simulink model "gm_uz_pmsm_model_9ph_21b_all_double_vnl"  (R2021b)
settings: Solver=FixedStepDiscrete  StartTime=0.0  StopTime=0.8  RelTol=1e-3
PreLoadFcn:
  | uz_pmsm_model_9ph_init_parameter
undefined symbols (not defined in the file or in its folder): a, b, c, friction_coefficient, inertia, k_i_d, k_i_q, k_p_d, k_p_q, Kpd, L_d, L_o1, L_o2, L_q, L_x1, L_x2, L_y1, L_y2, L_zero, polepair, psi_pm, R_1, static_friction_torque, Tnd, ts
libraries: hdlmdlgenlib x139, hdlsllib x90, dspsigops x21, simulink x17, slpidlib x2, spsAlphaBetaZerotodq0Lib x1, pid_lib x1, spsdq0toAlphaBetaZeroLib x1
(part 4 of 5)

== system gm_uz_pmsm_model_9ph_21b_all_double_vnl/uz_pmsm_model_9ph/Line-Line to Phase voltage/abc   to   alpha_beta_0 ==
  "a, b, c" : Inport  OutDataTypeStr=fixdt(1, 25, 12)  PortDimensions=[3]  SampleTime=1e-08
  Gain2 : Product  Inputs=**  OutDataTypeStr=fixdt(1, 43, 28)  SampleTime=1e-08
  Gain2_const : Constant  Value=0.6666717529296875  OutDataTypeStr=fixdt(1, 18, 16)  SampleTime=1e-08
  Gain2_out_dtc : DataTypeConversion  OutDataTypeStr=fixdt(1, 25, 12)  SampleTime=1e-08  SaturateOnIntegerOverflow=on
  Gain4_const : Constant  Value=[1;0;0.5;-0.5;0.86602783203125;0.5;-0.5;-0.86602783203125;0.5]  OutDataTypeStr=fixdt(1, 18, 16)  SampleTime=1e-08
  HwModeRegister{,1..3} (4 alike) : Delay  DelayLength=double(1)  InitialCondition=0  SampleTime=1e-08
  MMul_add_01 : Sum  OutDataTypeStr=fixdt(1, 25, 12)  SaturateOnIntegerOverflow=on  SampleTime=1e-08
  MMul_add_12 : Sum  OutDataTypeStr=fixdt(1, 25, 12)  SaturateOnIntegerOverflow=on  SampleTime=1e-08
  MMul_dot_product : Product  Inputs=**  OutDataTypeStr=fixdt(1, 43, 28)  SampleTime=1e-08
  MMul_dot_product_out_dtc : DataTypeConversion  OutDataTypeStr=fixdt(1, 25, 12)  SampleTime=1e-08  SaturateOnIntegerOverflow=on
  PipelineRegister : Delay  DelayLength=double(1)  InitialCondition=0  SampleTime=1e-08
  PipelineRegister1 : Delay  DelayLength=double(1)  InitialCondition=0  SampleTime=1e-08
  Reshape : Reshape  OutputDimensionality=Column vector (2-D)
  Row2Col_in0 : Reshape  OutputDimensionality=Column vector (2-D)
  Row2Col_in1 : Reshape  OutputDimensionality=Column vector (2-D)
  reshape_dotProduct : Reshape  OutputDimensionality=Customize  OutputDimensions=[3,3]
  reshape_mmulResult : Reshape  OutputDimensionality=Customize  OutputDimensions=[3,1]
  select_0 : Selector  NumberOfDimensions=2  SampleTime=1e-08  IndexOptions=Index vector (dialog),Select all  Indices=double(1),[]  OutputSizes=1
  select_1 : Selector  NumberOfDimensions=2  SampleTime=1e-08  IndexOptions=Index vector (dialog),Select all  Indices=double(2),[]  OutputSizes=1
  select_2 : Selector  NumberOfDimensions=2  SampleTime=1e-08  IndexOptions=Index vector (dialog),Select all  Indices=double(3),[]  OutputSizes=1
  select_indices0 : Selector  SampleTime=1e-08  IndexOptions=Index vector (dialog)  Indices=double([1 4 7 2 5 8 3 6 9])  OutputSizes=1
  select_indices1 : Selector  SampleTime=1e-08  IndexOptions=Index vector (dialog)  Indices=double([1 2 3 1 2 3 1 2 3])  OutputSizes=1
  t : Reshape  OutputDimensionality=Customize  OutputDimensions=[3,3]
  vectorized_in0 : Reshape  OutputDimensionality=Row vector (2-D)
  "alpha, beta, 0 " : Outport  SampleTime=1e-08
  wires:
  HwModeRegister3/1 -> Gain2/2
  HwModeRegister2/1 -> Gain2/1
  Gain2/1 -> PipelineRegister1/1
  HwModeRegister1/1 -> MMul_dot_product/2
  HwModeRegister/1 -> MMul_dot_product/1
  MMul_dot_product/1 -> PipelineRegister/1
  "a, b, c"/1 -> Reshape/1
  PipelineRegister1/1 -> Gain2_out_dtc/1
  PipelineRegister/1 -> MMul_dot_product_out_dtc/1
  Gain2_const/1 -> HwModeRegister3/1
  Gain4_const/1 -> t/1
  MMul_add_12/1 -> reshape_mmulResult/1
  select_2/1 -> MMul_add_12/2
  MMul_add_01/1 -> MMul_add_12/1
  select_1/1 -> MMul_add_01/2
  select_0/1 -> MMul_add_01/1
  reshape_dotProduct/1 -> select_0/1, select_1/1, select_2/1
  MMul_dot_product_out_dtc/1 -> reshape_dotProduct/1
  Row2Col_in1/1 -> HwModeRegister1/1
  Row2Col_in0/1 -> HwModeRegister/1
  select_indices1/1 -> Row2Col_in1/1
  select_indices0/1 -> Row2Col_in0/1
  vectorized_in0/1 -> select_indices0/1
  t/1 -> vectorized_in0/1
  Reshape/1 -> select_indices1/1
  reshape_mmulResult/1 -> HwModeRegister2/1
  Gain2_out_dtc/1 -> "alpha, beta, 0 "/1

== system gm_uz_pmsm_model_9ph_21b_all_double_vnl/uz_pmsm_model_9ph/Line-Line to Phase voltage/alpha_beta_0   to   abc ==
  "alpha, beta, 0  " : Inport  OutDataTypeStr=fixdt(1, 25, 12)  PortDimensions=[3]  SampleTime=1e-08
  Gain4_const : Constant  Value=[1;-0.5;-0.5;0;0.86602783203125;-0.86602783203125;1;1;1]  OutDataTypeStr=fixdt(1, 18, 16)  SampleTime=1e-08
  HwModeRegister : Delay  DelayLength=double(1)  InitialCondition=0  SampleTime=1e-08
  HwModeRegister1 : Delay  DelayLength=double(1)  InitialCondition=0  SampleTime=1e-08
  MMul_add_01 : Sum  OutDataTypeStr=fixdt(1, 25, 12)  SaturateOnIntegerOverflow=on  SampleTime=1e-08
  MMul_add_12 : Sum  OutDataTypeStr=fixdt(1, 25, 12)  SaturateOnIntegerOverflow=on  SampleTime=1e-08
  MMul_dot_product : Product  Inputs=**  OutDataTypeStr=fixdt(1, 43, 28)  SampleTime=1e-08
  MMul_dot_product_out_dtc : DataTypeConversion  OutDataTypeStr=fixdt(1, 25, 12)  SampleTime=1e-08  SaturateOnIntegerOverflow=on
  PipelineRegister : Delay  DelayLength=double(1)  InitialCondition=0  SampleTime=1e-08
  Reshape : Reshape  OutputDimensionality=Column vector (2-D)
  Row2Col_in0 : Reshape  OutputDimensionality=Column vector (2-D)
  Row2Col_in1 : Reshape  OutputDimensionality=Column vector (2-D)
  reshape_dotProduct : Reshape  OutputDimensionality=Customize  OutputDimensions=[3,3]
  reshape_mmulResult : Reshape  OutputDimensionality=Customize  OutputDimensions=[3,1]
  select_0 : Selector  NumberOfDimensions=2  SampleTime=1e-08  IndexOptions=Index vector (dialog),Select all  Indices=double(1),[]  OutputSizes=1
  select_1 : Selector  NumberOfDimensions=2  SampleTime=1e-08  IndexOptions=Index vector (dialog),Select all  Indices=double(2),[]  OutputSizes=1
  select_2 : Selector  NumberOfDimensions=2  SampleTime=1e-08  IndexOptions=Index vector (dialog),Select all  Indices=double(3),[]  OutputSizes=1
  select_indices0 : Selector  SampleTime=1e-08  IndexOptions=Index vector (dialog)  Indices=double([1 4 7 2 5 8 3 6 9])  OutputSizes=1
  select_indices1 : Selector  SampleTime=1e-08  IndexOptions=Index vector (dialog)  Indices=double([1 2 3 1 2 3 1 2 3])  OutputSizes=1
  t : Reshape  OutputDimensionality=Customize  OutputDimensions=[3,3]
  vectorized_in0 : Reshape  OutputDimensionality=Row vector (2-D)
  "a, b, c" : Outport  SampleTime=1e-08
  wires:
  HwModeRegister1/1 -> MMul_dot_product/2
  HwModeRegister/1 -> MMul_dot_product/1
  MMul_dot_product/1 -> PipelineRegister/1
  "alpha, beta, 0  "/1 -> Reshape/1
  PipelineRegister/1 -> MMul_dot_product_out_dtc/1
  Gain4_const/1 -> t/1
  MMul_add_12/1 -> reshape_mmulResult/1
  select_2/1 -> MMul_add_12/2
  MMul_add_01/1 -> MMul_add_12/1
  select_1/1 -> MMul_add_01/2
  select_0/1 -> MMul_add_01/1
  reshape_dotProduct/1 -> select_0/1, select_1/1, select_2/1
  MMul_dot_product_out_dtc/1 -> reshape_dotProduct/1
  Row2Col_in1/1 -> HwModeRegister1/1
  Row2Col_in0/1 -> HwModeRegister/1
  select_indices1/1 -> Row2Col_in1/1
  select_indices0/1 -> Row2Col_in0/1
  vectorized_in0/1 -> select_indices0/1
  t/1 -> vectorized_in0/1
  Reshape/1 -> select_indices1/1
  reshape_mmulResult/1 -> "a, b, c"/1

== system gm_uz_pmsm_model_9ph_21b_all_double_vnl/uz_pmsm_model_9ph/Line-Line to Phase voltage1/abc   to   alpha_beta_0 ==
  "a, b, c" : Inport  OutDataTypeStr=fixdt(1, 25, 12)  PortDimensions=[3]  SampleTime=1e-08
  Gain2 : Product  Inputs=**  OutDataTypeStr=fixdt(1, 43, 28)  SampleTime=1e-08
  Gain2_const : Constant  Value=0.6666717529296875  OutDataTypeStr=fixdt(1, 18, 16)  SampleTime=1e-08
  Gain2_out_dtc : DataTypeConversion  OutDataTypeStr=fixdt(1, 25, 12)  SampleTime=1e-08  SaturateOnIntegerOverflow=on
  Gain4_const : Constant  Value=[1;0;0.5;-0.5;0.86602783203125;0.5;-0.5;-0.86602783203125;0.5]  OutDataTypeStr=fixdt(1, 18, 16)  SampleTime=1e-08
  HwModeRegister{,1..3} (4 alike) : Delay  DelayLength=double(1)  InitialCondition=0  SampleTime=1e-08
  MMul_add_01 : Sum  OutDataTypeStr=fixdt(1, 25, 12)  SaturateOnIntegerOverflow=on  SampleTime=1e-08
  MMul_add_12 : Sum  OutDataTypeStr=fixdt(1, 25, 12)  SaturateOnIntegerOverflow=on  SampleTime=1e-08
  MMul_dot_product : Product  Inputs=**  OutDataTypeStr=fixdt(1, 43, 28)  SampleTime=1e-08
  MMul_dot_product_out_dtc : DataTypeConversion  OutDataTypeStr=fixdt(1, 25, 12)  SampleTime=1e-08  SaturateOnIntegerOverflow=on
  PipelineRegister : Delay  DelayLength=double(1)  InitialCondition=0  SampleTime=1e-08
  PipelineRegister1 : Delay  DelayLength=double(1)  InitialCondition=0  SampleTime=1e-08
  Reshape : Reshape  OutputDimensionality=Column vector (2-D)
  Row2Col_in0 : Reshape  OutputDimensionality=Column vector (2-D)
  Row2Col_in1 : Reshape  OutputDimensionality=Column vector (2-D)
  reshape_dotProduct : Reshape  OutputDimensionality=Customize  OutputDimensions=[3,3]
  reshape_mmulResult : Reshape  OutputDimensionality=Customize  OutputDimensions=[3,1]
  select_0 : Selector  NumberOfDimensions=2  SampleTime=1e-08  IndexOptions=Index vector (dialog),Select all  Indices=double(1),[]  OutputSizes=1
  select_1 : Selector  NumberOfDimensions=2  SampleTime=1e-08  IndexOptions=Index vector (dialog),Select all  Indices=double(2),[]  OutputSizes=1
  select_2 : Selector  NumberOfDimensions=2  SampleTime=1e-08  IndexOptions=Index vector (dialog),Select all  Indices=double(3),[]  OutputSizes=1
  select_indices0 : Selector  SampleTime=1e-08  IndexOptions=Index vector (dialog)  Indices=double([1 4 7 2 5 8 3 6 9])  OutputSizes=1
  select_indices1 : Selector  SampleTime=1e-08  IndexOptions=Index vector (dialog)  Indices=double([1 2 3 1 2 3 1 2 3])  OutputSizes=1
  t : Reshape  OutputDimensionality=Customize  OutputDimensions=[3,3]
  vectorized_in0 : Reshape  OutputDimensionality=Row vector (2-D)
  "alpha, beta, 0 " : Outport  SampleTime=1e-08
  wires:
  HwModeRegister3/1 -> Gain2/2
  HwModeRegister2/1 -> Gain2/1
  Gain2/1 -> PipelineRegister1/1
  HwModeRegister1/1 -> MMul_dot_product/2
  HwModeRegister/1 -> MMul_dot_product/1
  MMul_dot_product/1 -> PipelineRegister/1
  "a, b, c"/1 -> Reshape/1
  PipelineRegister1/1 -> Gain2_out_dtc/1
  PipelineRegister/1 -> MMul_dot_product_out_dtc/1
  Gain2_const/1 -> HwModeRegister3/1
  Gain4_const/1 -> t/1
  MMul_add_12/1 -> reshape_mmulResult/1
  select_2/1 -> MMul_add_12/2
  MMul_add_01/1 -> MMul_add_12/1
  select_1/1 -> MMul_add_01/2
  select_0/1 -> MMul_add_01/1
  reshape_dotProduct/1 -> select_0/1, select_1/1, select_2/1
  MMul_dot_product_out_dtc/1 -> reshape_dotProduct/1
  Row2Col_in1/1 -> HwModeRegister1/1
  Row2Col_in0/1 -> HwModeRegister/1
  select_indices1/1 -> Row2Col_in1/1
  select_indices0/1 -> Row2Col_in0/1
  vectorized_in0/1 -> select_indices0/1
  t/1 -> vectorized_in0/1
  Reshape/1 -> select_indices1/1
  reshape_mmulResult/1 -> HwModeRegister2/1
  Gain2_out_dtc/1 -> "alpha, beta, 0 "/1

== system gm_uz_pmsm_model_9ph_21b_all_double_vnl/uz_pmsm_model_9ph/Line-Line to Phase voltage1/alpha_beta_0   to   abc ==
  "alpha, beta, 0  " : Inport  OutDataTypeStr=fixdt(1, 25, 12)  PortDimensions=[3]  SampleTime=1e-08
  Gain4_const : Constant  Value=[1;-0.5;-0.5;0;0.86602783203125;-0.86602783203125;1;1;1]  OutDataTypeStr=fixdt(1, 18, 16)  SampleTime=1e-08
  HwModeRegister : Delay  DelayLength=double(1)  InitialCondition=0  SampleTime=1e-08
  HwModeRegister1 : Delay  DelayLength=double(1)  InitialCondition=0  SampleTime=1e-08
  MMul_add_01 : Sum  OutDataTypeStr=fixdt(1, 25, 12)  SaturateOnIntegerOverflow=on  SampleTime=1e-08
  MMul_add_12 : Sum  OutDataTypeStr=fixdt(1, 25, 12)  SaturateOnIntegerOverflow=on  SampleTime=1e-08
  MMul_dot_product : Product  Inputs=**  OutDataTypeStr=fixdt(1, 43, 28)  SampleTime=1e-08
  MMul_dot_product_out_dtc : DataTypeConversion  OutDataTypeStr=fixdt(1, 25, 12)  SampleTime=1e-08  SaturateOnIntegerOverflow=on
  PipelineRegister : Delay  DelayLength=double(1)  InitialCondition=0  SampleTime=1e-08
  Reshape : Reshape  OutputDimensionality=Column vector (2-D)
  Row2Col_in0 : Reshape  OutputDimensionality=Column vector (2-D)
  Row2Col_in1 : Reshape  OutputDimensionality=Column vector (2-D)
  reshape_dotProduct : Reshape  OutputDimensionality=Customize  OutputDimensions=[3,3]
  reshape_mmulResult : Reshape  OutputDimensionality=Customize  OutputDimensions=[3,1]
  select_0 : Selector  NumberOfDimensions=2  SampleTime=1e-08  IndexOptions=Index vector (dialog),Select all  Indices=double(1),[]  OutputSizes=1
  select_1 : Selector  NumberOfDimensions=2  SampleTime=1e-08  IndexOptions=Index vector (dialog),Select all  Indices=double(2),[]  OutputSizes=1
  select_2 : Selector  NumberOfDimensions=2  SampleTime=1e-08  IndexOptions=Index vector (dialog),Select all  Indices=double(3),[]  OutputSizes=1
  select_indices0 : Selector  SampleTime=1e-08  IndexOptions=Index vector (dialog)  Indices=double([1 4 7 2 5 8 3 6 9])  OutputSizes=1
  select_indices1 : Selector  SampleTime=1e-08  IndexOptions=Index vector (dialog)  Indices=double([1 2 3 1 2 3 1 2 3])  OutputSizes=1
  t : Reshape  OutputDimensionality=Customize  OutputDimensions=[3,3]
  vectorized_in0 : Reshape  OutputDimensionality=Row vector (2-D)
  "a, b, c" : Outport  SampleTime=1e-08
  wires:
  HwModeRegister1/1 -> MMul_dot_product/2
  HwModeRegister/1 -> MMul_dot_product/1
  MMul_dot_product/1 -> PipelineRegister/1
  "alpha, beta, 0  "/1 -> Reshape/1
  PipelineRegister/1 -> MMul_dot_product_out_dtc/1
  Gain4_const/1 -> t/1
  MMul_add_12/1 -> reshape_mmulResult/1
  select_2/1 -> MMul_add_12/2
  MMul_add_01/1 -> MMul_add_12/1
  select_1/1 -> MMul_add_01/2
  select_0/1 -> MMul_add_01/1
  reshape_dotProduct/1 -> select_0/1, select_1/1, select_2/1
  MMul_dot_product_out_dtc/1 -> reshape_dotProduct/1
  Row2Col_in1/1 -> HwModeRegister1/1
  Row2Col_in0/1 -> HwModeRegister/1
  select_indices1/1 -> Row2Col_in1/1
  select_indices0/1 -> Row2Col_in0/1
  vectorized_in0/1 -> select_indices0/1
  t/1 -> vectorized_in0/1
  Reshape/1 -> select_indices1/1
  reshape_mmulResult/1 -> "a, b, c"/1

== system gm_uz_pmsm_model_9ph_21b_all_double_vnl/uz_pmsm_model_9ph/Line-Line to Phase voltage2/abc   to   alpha_beta_0 ==
  "a, b, c" : Inport  OutDataTypeStr=fixdt(1, 25, 12)  PortDimensions=[3]  SampleTime=1e-08
  Gain2 : Product  Inputs=**  OutDataTypeStr=fixdt(1, 43, 28)  SampleTime=1e-08
  Gain2_const : Constant  Value=0.6666717529296875  OutDataTypeStr=fixdt(1, 18, 16)  SampleTime=1e-08
  Gain2_out_dtc : DataTypeConversion  OutDataTypeStr=fixdt(1, 25, 12)  SampleTime=1e-08  SaturateOnIntegerOverflow=on
  Gain4_const : Constant  Value=[1;0;0.5;-0.5;0.86602783203125;0.5;-0.5;-0.86602783203125;0.5]  OutDataTypeStr=fixdt(1, 18, 16)  SampleTime=1e-08
  HwModeRegister{,1..3} (4 alike) : Delay  DelayLength=double(1)  InitialCondition=0  SampleTime=1e-08
  MMul_add_01 : Sum  OutDataTypeStr=fixdt(1, 25, 12)  SaturateOnIntegerOverflow=on  SampleTime=1e-08
  MMul_add_12 : Sum  OutDataTypeStr=fixdt(1, 25, 12)  SaturateOnIntegerOverflow=on  SampleTime=1e-08
  MMul_dot_product : Product  Inputs=**  OutDataTypeStr=fixdt(1, 43, 28)  SampleTime=1e-08
  MMul_dot_product_out_dtc : DataTypeConversion  OutDataTypeStr=fixdt(1, 25, 12)  SampleTime=1e-08  SaturateOnIntegerOverflow=on
  PipelineRegister : Delay  DelayLength=double(1)  InitialCondition=0  SampleTime=1e-08
  PipelineRegister1 : Delay  DelayLength=double(1)  InitialCondition=0  SampleTime=1e-08
  Reshape : Reshape  OutputDimensionality=Column vector (2-D)
  Row2Col_in0 : Reshape  OutputDimensionality=Column vector (2-D)
  Row2Col_in1 : Reshape  OutputDimensionality=Column vector (2-D)
  reshape_dotProduct : Reshape  OutputDimensionality=Customize  OutputDimensions=[3,3]
  reshape_mmulResult : Reshape  OutputDimensionality=Customize  OutputDimensions=[3,1]
  select_0 : Selector  NumberOfDimensions=2  SampleTime=1e-08  IndexOptions=Index vector (dialog),Select all  Indices=double(1),[]  OutputSizes=1
  select_1 : Selector  NumberOfDimensions=2  SampleTime=1e-08  IndexOptions=Index vector (dialog),Select all  Indices=double(2),[]  OutputSizes=1
  select_2 : Selector  NumberOfDimensions=2  SampleTime=1e-08  IndexOptions=Index vector (dialog),Select all  Indices=double(3),[]  OutputSizes=1
  select_indices0 : Selector  SampleTime=1e-08  IndexOptions=Index vector (dialog)  Indices=double([1 4 7 2 5 8 3 6 9])  OutputSizes=1
  select_indices1 : Selector  SampleTime=1e-08  IndexOptions=Index vector (dialog)  Indices=double([1 2 3 1 2 3 1 2 3])  OutputSizes=1
  t : Reshape  OutputDimensionality=Customize  OutputDimensions=[3,3]
  vectorized_in0 : Reshape  OutputDimensionality=Row vector (2-D)
  "alpha, beta, 0 " : Outport  SampleTime=1e-08
  wires:
  HwModeRegister3/1 -> Gain2/2
  HwModeRegister2/1 -> Gain2/1
  Gain2/1 -> PipelineRegister1/1
  HwModeRegister1/1 -> MMul_dot_product/2
  HwModeRegister/1 -> MMul_dot_product/1
  MMul_dot_product/1 -> PipelineRegister/1
  "a, b, c"/1 -> Reshape/1
  PipelineRegister1/1 -> Gain2_out_dtc/1
  PipelineRegister/1 -> MMul_dot_product_out_dtc/1
  Gain2_const/1 -> HwModeRegister3/1
  Gain4_const/1 -> t/1
  MMul_add_12/1 -> reshape_mmulResult/1
  select_2/1 -> MMul_add_12/2
  MMul_add_01/1 -> MMul_add_12/1
  select_1/1 -> MMul_add_01/2
  select_0/1 -> MMul_add_01/1
  reshape_dotProduct/1 -> select_0/1, select_1/1, select_2/1
  MMul_dot_product_out_dtc/1 -> reshape_dotProduct/1
  Row2Col_in1/1 -> HwModeRegister1/1
  Row2Col_in0/1 -> HwModeRegister/1
  select_indices1/1 -> Row2Col_in1/1
  select_indices0/1 -> Row2Col_in0/1
  vectorized_in0/1 -> select_indices0/1
  t/1 -> vectorized_in0/1
  Reshape/1 -> select_indices1/1
  reshape_mmulResult/1 -> HwModeRegister2/1
  Gain2_out_dtc/1 -> "alpha, beta, 0 "/1

== system gm_uz_pmsm_model_9ph_21b_all_double_vnl/uz_pmsm_model_9ph/Line-Line to Phase voltage2/alpha_beta_0   to   abc ==
  "alpha, beta, 0  " : Inport  OutDataTypeStr=fixdt(1, 25, 12)  PortDimensions=[3]  SampleTime=1e-08
  Gain4_const : Constant  Value=[1;-0.5;-0.5;0;0.86602783203125;-0.86602783203125;1;1;1]  OutDataTypeStr=fixdt(1, 18, 16)  SampleTime=1e-08
  HwModeRegister : Delay  DelayLength=double(1)  InitialCondition=0  SampleTime=1e-08
  HwModeRegister1 : Delay  DelayLength=double(1)  InitialCondition=0  SampleTime=1e-08
  MMul_add_01 : Sum  OutDataTypeStr=fixdt(1, 25, 12)  SaturateOnIntegerOverflow=on  SampleTime=1e-08
  MMul_add_12 : Sum  OutDataTypeStr=fixdt(1, 25, 12)  SaturateOnIntegerOverflow=on  SampleTime=1e-08
  MMul_dot_product : Product  Inputs=**  OutDataTypeStr=fixdt(1, 43, 28)  SampleTime=1e-08
  MMul_dot_product_out_dtc : DataTypeConversion  OutDataTypeStr=fixdt(1, 25, 12)  SampleTime=1e-08  SaturateOnIntegerOverflow=on
  PipelineRegister : Delay  DelayLength=double(1)  InitialCondition=0  SampleTime=1e-08
  Reshape : Reshape  OutputDimensionality=Column vector (2-D)
  Row2Col_in0 : Reshape  OutputDimensionality=Column vector (2-D)
  Row2Col_in1 : Reshape  OutputDimensionality=Column vector (2-D)
  reshape_dotProduct : Reshape  OutputDimensionality=Customize  OutputDimensions=[3,3]
  reshape_mmulResult : Reshape  OutputDimensionality=Customize  OutputDimensions=[3,1]
  select_0 : Selector  NumberOfDimensions=2  SampleTime=1e-08  IndexOptions=Index vector (dialog),Select all  Indices=double(1),[]  OutputSizes=1
  select_1 : Selector  NumberOfDimensions=2  SampleTime=1e-08  IndexOptions=Index vector (dialog),Select all  Indices=double(2),[]  OutputSizes=1
  select_2 : Selector  NumberOfDimensions=2  SampleTime=1e-08  IndexOptions=Index vector (dialog),Select all  Indices=double(3),[]  OutputSizes=1
  select_indices0 : Selector  SampleTime=1e-08  IndexOptions=Index vector (dialog)  Indices=double([1 4 7 2 5 8 3 6 9])  OutputSizes=1
  select_indices1 : Selector  SampleTime=1e-08  IndexOptions=Index vector (dialog)  Indices=double([1 2 3 1 2 3 1 2 3])  OutputSizes=1
  t : Reshape  OutputDimensionality=Customize  OutputDimensions=[3,3]
  vectorized_in0 : Reshape  OutputDimensionality=Row vector (2-D)
  "a, b, c" : Outport  SampleTime=1e-08
  wires:
  HwModeRegister1/1 -> MMul_dot_product/2
  HwModeRegister/1 -> MMul_dot_product/1
  MMul_dot_product/1 -> PipelineRegister/1
  "alpha, beta, 0  "/1 -> Reshape/1
  PipelineRegister/1 -> MMul_dot_product_out_dtc/1
  Gain4_const/1 -> t/1
  MMul_add_12/1 -> reshape_mmulResult/1
  select_2/1 -> MMul_add_12/2
  MMul_add_01/1 -> MMul_add_12/1
  select_1/1 -> MMul_add_01/2
  select_0/1 -> MMul_add_01/1
  reshape_dotProduct/1 -> select_0/1, select_1/1, select_2/1
  MMul_dot_product_out_dtc/1 -> reshape_dotProduct/1
  Row2Col_in1/1 -> HwModeRegister1/1
  Row2Col_in0/1 -> HwModeRegister/1
  select_indices1/1 -> Row2Col_in1/1
  select_indices0/1 -> Row2Col_in0/1
  vectorized_in0/1 -> select_indices0/1
  t/1 -> vectorized_in0/1
  Reshape/1 -> select_indices1/1
  reshape_mmulResult/1 -> "a, b, c"/1

== system gm_uz_pmsm_model_9ph_21b_all_double_vnl/uz_pmsm_model_9ph/Transformation/Add ==
  In1 : Inport
  In2 : Inport  Port=2
  Add : Sum  OutDataTypeStr=single  SampleTime=1e-08
  Add_pd1 : Delay  DelayLength=6
  Out1 : Outport
  wires:
  Add_pd1/1 -> Out1/1
  Add/1 -> Add_pd1/1
  In2/1 -> Add/2
  In1/1 -> Add/1

== system gm_uz_pmsm_model_9ph_21b_all_double_vnl/uz_pmsm_model_9ph/Transformation/Add1 ==
  In1 : Inport
  In2 : Inport  Port=2
  Add1 : Sum  Inputs=+-  OutDataTypeStr=single  SampleTime=1e-08
  Add1_pd1 : Delay  DelayLength=6
  Out1 : Outport
  wires:
  Add1_pd1/1 -> Out1/1
  Add1/1 -> Add1_pd1/1
  In2/1 -> Add1/2
  In1/1 -> Add1/1

== system gm_uz_pmsm_model_9ph_21b_all_double_vnl/uz_pmsm_model_9ph/Transformation/Data Type Conversion39 ==
  In1 : Inport
  Data Type Conversion39 : DataTypeConversion  OutDataTypeStr=single  RndMeth=Nearest  SampleTime=1e-08
  Data Type Conversion39_pd1 : Delay  DelayLength=6
  Out1 : Outport
  wires:
  Data Type Conversion39_pd1/1 -> Out1/1
  Data Type Conversion39/1 -> Data Type Conversion39_pd1/1
  In1/1 -> Data Type Conversion39/1

== system gm_uz_pmsm_model_9ph_21b_all_double_vnl/uz_pmsm_model_9ph/Transformation/Divide ==
  In1 : Inport
  In2 : Inport  Port=2
  Divide : Product  Inputs=**  OutDataTypeStr=single  SampleTime=1e-08
  Divide_pd1 : Delay  DelayLength=6
  Out1 : Outport
  wires:
  Divide_pd1/1 -> Out1/1
  Divide/1 -> Divide_pd1/1
  In2/1 -> Divide/2
  In1/1 -> Divide/1

== system gm_uz_pmsm_model_9ph_21b_all_double_vnl/uz_pmsm_model_9ph/Transformation/Divide1 ==
  In1 : Inport
  In2 : Inport  Port=2
  Divide1 : Product  Inputs=**  OutDataTypeStr=single  SampleTime=1e-08
  Divide1_pd1 : Delay  DelayLength=6
  Out1 : Outport
  wires:
  Divide1_pd1/1 -> Out1/1
  Divide1/1 -> Divide1_pd1/1
  In2/1 -> Divide1/2
  In1/1 -> Divide1/1

== system gm_uz_pmsm_model_9ph_21b_all_double_vnl/uz_pmsm_model_9ph/Transformation/Divide2 ==
  In1 : Inport
  In2 : Inport  Port=2
  Divide2 : Product  Inputs=**  OutDataTypeStr=single  SampleTime=1e-08
  Divide2_pd1 : Delay  DelayLength=6
  Out1 : Outport
  wires:
  Divide2_pd1/1 -> Out1/1
  Divide2/1 -> Divide2_pd1/1
  In2/1 -> Divide2/2
  In1/1 -> Divide2/1

== system gm_uz_pmsm_model_9ph_21b_all_double_vnl/uz_pmsm_model_9ph/Transformation/Divide3 ==
  In1 : Inport
  In2 : Inport  Port=2
  Divide3 : Product  Inputs=**  OutDataTypeStr=single  SampleTime=1e-08
  Divide3_pd1 : Delay  DelayLength=6
  Out1 : Outport
  wires:
  Divide3_pd1/1 -> Out1/1
  Divide3/1 -> Divide3_pd1/1
  In2/1 -> Divide3/2
  In1/1 -> Divide3/1

== system gm_uz_pmsm_model_9ph_21b_all_double_vnl/uz_pmsm_model_9ph/Transformation/t3 ==
  in0 : Inport
  ColVec1 : Selector  NumberOfDimensions=2  IndexOptions=Select all,Index vector (dialog)  Indices=1,1  OutputSizes=1,1
  ColVec2 : Selector  NumberOfDimensions=2  IndexOptions=Select all,Index vector (dialog)  Indices=1,2  OutputSizes=1,1
  ColVec3 : Selector  NumberOfDimensions=2  IndexOptions=Select all,Index vector (dialog)  Indices=1,3  OutputSizes=1,1
  ColVec4 : Selector  NumberOfDimensions=2  IndexOptions=Select all,Index vector (dialog)  Indices=1,4  OutputSizes=1,1
  ColVec5 : Selector  NumberOfDimensions=2  IndexOptions=Select all,Index vector (dialog)  Indices=1,5  OutputSizes=1,1
  ColVec6 : Selector  NumberOfDimensions=2  IndexOptions=Select all,Index vector (dialog)  Indices=1,6  OutputSizes=1,1
  ColVec7 : Selector  NumberOfDimensions=2  IndexOptions=Select all,Index vector (dialog)  Indices=1,7  OutputSizes=1,1
  ColVec8 : Selector  NumberOfDimensions=2  IndexOptions=Select all,Index vector (dialog)  Indices=1,8  OutputSizes=1,1
  ColVec9 : Selector  NumberOfDimensions=2  IndexOptions=Select all,Index vector (dialog)  Indices=1,9  OutputSizes=1,1
  out0 : Outport
  out1 : Outport  Port=2
  out2 : Outport  Port=3
  out3 : Outport  Port=4
  out4 : Outport  Port=5
  out5 : Outport  Port=6
  out6 : Outport  Port=7
  out7 : Outport  Port=8
  out8 : Outport  Port=9
  wires:
  ColVec9/1 -> out8/1
  ColVec8/1 -> out7/1
  ColVec7/1 -> out6/1
  ColVec6/1 -> out5/1
  ColVec5/1 -> out4/1
  ColVec4/1 -> out3/1
  ColVec3/1 -> out2/1
  ColVec2/1 -> out1/1
  ColVec1/1 -> out0/1
  in0/1 -> ColVec9/1, ColVec8/1, ColVec7/1, ColVec6/1, ColVec5/1, ColVec4/1, ColVec3/1, ColVec2/1, ColVec1/1

== system gm_uz_pmsm_model_9ph_21b_all_double_vnl/uz_pmsm_model_9ph/Transformation1/Add ==
  In1 : Inport
  In2 : Inport  Port=2
  Add : Sum  Inputs=+-  OutDataTypeStr=single  SampleTime=1e-08
  Add_pd1 : Delay  DelayLength=6
  Out1 : Outport
  wires:
  Add_pd1/1 -> Out1/1
  Add/1 -> Add_pd1/1
  In2/1 -> Add/2
  In1/1 -> Add/1

== system gm_uz_pmsm_model_9ph_21b_all_double_vnl/uz_pmsm_model_9ph/Transformation1/Add1 ==
  In1 : Inport
  In2 : Inport  Port=2
  Add1 : Sum  OutDataTypeStr=single  SampleTime=1e-08
  Add1_pd1 : Delay  DelayLength=6
  Out1 : Outport
  wires:
  Add1_pd1/1 -> Out1/1
  Add1/1 -> Add1_pd1/1
  In2/1 -> Add1/2
  In1/1 -> Add1/1

== system gm_uz_pmsm_model_9ph_21b_all_double_vnl/uz_pmsm_model_9ph/Transformation1/Data Type Conversion28 ==
  In1 : Inport
  Data Type Conversion28 : DataTypeConversion  OutDataTypeStr=fixdt(1, 25, 12)  RndMeth=Nearest  SampleTime=1e-08
  Data Type Conversion28_pd1 : Delay  DelayLength=6
  Out1 : Outport
  wires:
  Data Type Conversion28_pd1/1 -> Out1/1
  Data Type Conversion28/1 -> Data Type Conversion28_pd1/1
  In1/1 -> Data Type Conversion28/1

== system gm_uz_pmsm_model_9ph_21b_all_double_vnl/uz_pmsm_model_9ph/Transformation1/Divide ==
  In1 : Inport
  In2 : Inport  Port=2
  Divide : Product  Inputs=**  OutDataTypeStr=single  SampleTime=1e-08
  Divide_pd1 : Delay  DelayLength=6
  Out1 : Outport
  wires:
  Divide_pd1/1 -> Out1/1
  Divide/1 -> Divide_pd1/1
  In2/1 -> Divide/2
  In1/1 -> Divide/1

== system gm_uz_pmsm_model_9ph_21b_all_double_vnl/uz_pmsm_model_9ph/Transformation1/Divide1 ==
  In1 : Inport
  In2 : Inport  Port=2
  Divide1 : Product  Inputs=**  OutDataTypeStr=single  SampleTime=1e-08
  Divide1_pd1 : Delay  DelayLength=6
  Out1 : Outport
  wires:
  Divide1_pd1/1 -> Out1/1
  Divide1/1 -> Divide1_pd1/1
  In2/1 -> Divide1/2
  In1/1 -> Divide1/1

== system gm_uz_pmsm_model_9ph_21b_all_double_vnl/uz_pmsm_model_9ph/Transformation1/Divide2 ==
  In1 : Inport
  In2 : Inport  Port=2
  Divide2 : Product  Inputs=**  OutDataTypeStr=single  SampleTime=1e-08
  Divide2_pd1 : Delay  DelayLength=6
  Out1 : Outport
  wires:
  Divide2_pd1/1 -> Out1/1
  Divide2/1 -> Divide2_pd1/1
  In2/1 -> Divide2/2
  In1/1 -> Divide2/1

== system gm_uz_pmsm_model_9ph_21b_all_double_vnl/uz_pmsm_model_9ph/Transformation1/Divide3 ==
  In1 : Inport
  In2 : Inport  Port=2
  Divide3 : Product  Inputs=**  OutDataTypeStr=single  SampleTime=1e-08
  Divide3_pd1 : Delay  DelayLength=6
  Out1 : Outport
  wires:
  Divide3_pd1/1 -> Out1/1
  Divide3/1 -> Divide3_pd1/1
  In2/1 -> Divide3/2
  In1/1 -> Divide3/1

== system gm_uz_pmsm_model_9ph_21b_all_double_vnl/uz_pmsm_model_9ph/Transformation1/Transformation1_MAC ==
  in0 : Inport  OutDataTypeStr=fixdt(1, 18, 16)  PortDimensions=[9 1]  SampleTime=1e-08
  in1 : Inport  Port=2  OutDataTypeStr=fixdt(1, 25, 12)  PortDimensions=[9]  SampleTime=1e-08
  globalSchedule : EnablePort  OutDataTypeStr=boolean
  PipelineRegister : Delay  DelayLength=double(8)  InitialCondition=0
  t : hdlsllib/HDL Operations/Multiply-Accumulate  opMode=Vector  initValueSetting=Dialog  initValue=0  initValueSetting2=Dialog  initValue2=0  initValueSetting3=Dialog  initValue3=0  num_samples=2  RndMeth2=Floor  RndMeth3=Floor  OutDataTypeStr=fixdt(1, 25, 12)  datatype2=Inherit: Inherit via back propagation  datatype3=Inherit: Inherit via back propagation  validOut=on  endInandOut=on  startOut=on  countOut=on  dim=-1  DoSatur=off  parallel=off
      settings: SourceProductBaseCode=SL
  out0 : Outport  OutDataTypeStr=fixdt(1, 25, 12)  SampleTime=1e-08  InitialOutput=0
  wires:
  t/1 -> PipelineRegister/1
  in1/1 -> t/2
  in0/1 -> t/1
  PipelineRegister/1 -> out0/1

== system gm_uz_pmsm_model_9ph_21b_all_double_vnl/uz_pmsm_model_9ph/Transformation1/Transformation1_MAC1 ==
  in0 : Inport  OutDataTypeStr=fixdt(1, 18, 16)  PortDimensions=[9 1]  SampleTime=1e-08
  in1 : Inport  Port=2  OutDataTypeStr=fixdt(1, 25, 12)  PortDimensions=[9]  SampleTime=1e-08
  globalSchedule : EnablePort  OutDataTypeStr=boolean
  PipelineRegister : Delay  DelayLength=double(8)  InitialCondition=0
  t : hdlsllib/HDL Operations/Multiply-Accumulate  opMode=Vector  initValueSetting=Dialog  initValue=0  initValueSetting2=Dialog  initValue2=0  initValueSetting3=Dialog  initValue3=0  num_samples=2  RndMeth2=Floor  RndMeth3=Floor  OutDataTypeStr=fixdt(1, 25, 12)  datatype2=Inherit: Inherit via back propagation  datatype3=Inherit: Inherit via back propagation  validOut=on  endInandOut=on  startOut=on  countOut=on  dim=-1  DoSatur=off  parallel=off
      settings: SourceProductBaseCode=SL
  out0 : Outport  OutDataTypeStr=fixdt(1, 25, 12)  SampleTime=1e-08  InitialOutput=0
  wires:
  t/1 -> PipelineRegister/1
  in1/1 -> t/2
  in0/1 -> t/1
  PipelineRegister/1 -> out0/1

== system gm_uz_pmsm_model_9ph_21b_all_double_vnl/uz_pmsm_model_9ph/Transformation1/Transformation1_MAC2 ==
  in0 : Inport  OutDataTypeStr=fixdt(1, 18, 16)  PortDimensions=[9 1]  SampleTime=1e-08
  in1 : Inport  Port=2  OutDataTypeStr=fixdt(1, 25, 12)  PortDimensions=[9]  SampleTime=1e-08
  globalSchedule : EnablePort  OutDataTypeStr=boolean
  PipelineRegister : Delay  DelayLength=double(8)  InitialCondition=0
  t : hdlsllib/HDL Operations/Multiply-Accumulate  opMode=Vector  initValueSetting=Dialog  initValue=0  initValueSetting2=Dialog  initValue2=0  initValueSetting3=Dialog  initValue3=0  num_samples=2  RndMeth2=Floor  RndMeth3=Floor  OutDataTypeStr=fixdt(1, 25, 12)  datatype2=Inherit: Inherit via back propagation  datatype3=Inherit: Inherit via back propagation  validOut=on  endInandOut=on  startOut=on  countOut=on  dim=-1  DoSatur=off  parallel=off
      settings: SourceProductBaseCode=SL
  out0 : Outport  OutDataTypeStr=fixdt(1, 25, 12)  SampleTime=1e-08  InitialOutput=0
  wires:
  t/1 -> PipelineRegister/1
  in1/1 -> t/2
  in0/1 -> t/1
  PipelineRegister/1 -> out0/1

== system gm_uz_pmsm_model_9ph_21b_all_double_vnl/uz_pmsm_model_9ph/Transformation1/Transformation1_MAC3 ==
  in0 : Inport  OutDataTypeStr=fixdt(1, 18, 16)  PortDimensions=[9 1]  SampleTime=1e-08
  in1 : Inport  Port=2  OutDataTypeStr=fixdt(1, 25, 12)  PortDimensions=[9]  SampleTime=1e-08
  globalSchedule : EnablePort  OutDataTypeStr=boolean
  PipelineRegister : Delay  DelayLength=double(8)  InitialCondition=0
  t : hdlsllib/HDL Operations/Multiply-Accumulate  opMode=Vector  initValueSetting=Dialog  initValue=0  initValueSetting2=Dialog  initValue2=0  initValueSetting3=Dialog  initValue3=0  num_samples=2  RndMeth2=Floor  RndMeth3=Floor  OutDataTypeStr=fixdt(1, 25, 12)  datatype2=Inherit: Inherit via back propagation  datatype3=Inherit: Inherit via back propagation  validOut=on  endInandOut=on  startOut=on  countOut=on  dim=-1  DoSatur=off  parallel=off
      settings: SourceProductBaseCode=SL
  out0 : Outport  OutDataTypeStr=fixdt(1, 25, 12)  SampleTime=1e-08  InitialOutput=0
  wires:
  t/1 -> PipelineRegister/1
  in1/1 -> t/2
  in0/1 -> t/1
  PipelineRegister/1 -> out0/1

== system gm_uz_pmsm_model_9ph_21b_all_double_vnl/uz_pmsm_model_9ph/Transformation1/Transformation1_MAC4 ==
  in0 : Inport  OutDataTypeStr=fixdt(1, 18, 16)  PortDimensions=[9 1]  SampleTime=1e-08
  in1 : Inport  Port=2  OutDataTypeStr=fixdt(1, 25, 12)  PortDimensions=[9]  SampleTime=1e-08
  globalSchedule : EnablePort  OutDataTypeStr=boolean
  PipelineRegister : Delay  DelayLength=double(8)  InitialCondition=0
  t : hdlsllib/HDL Operations/Multiply-Accumulate  opMode=Vector  initValueSetting=Dialog  initValue=0  initValueSetting2=Dialog  initValue2=0  initValueSetting3=Dialog  initValue3=0  num_samples=2  RndMeth2=Floor  RndMeth3=Floor  OutDataTypeStr=fixdt(1, 25, 12)  datatype2=Inherit: Inherit via back propagation  datatype3=Inherit: Inherit via back propagation  validOut=on  endInandOut=on  startOut=on  countOut=on  dim=-1  DoSatur=off  parallel=off
      settings: SourceProductBaseCode=SL
  out0 : Outport  OutDataTypeStr=fixdt(1, 25, 12)  SampleTime=1e-08  InitialOutput=0
  wires:
  t/1 -> PipelineRegister/1
  in1/1 -> t/2
  in0/1 -> t/1
  PipelineRegister/1 -> out0/1

== system gm_uz_pmsm_model_9ph_21b_all_double_vnl/uz_pmsm_model_9ph/Transformation1/Transformation1_MAC5 ==
  in0 : Inport  OutDataTypeStr=fixdt(1, 18, 16)  PortDimensions=[9 1]  SampleTime=1e-08
  in1 : Inport  Port=2  OutDataTypeStr=fixdt(1, 25, 12)  PortDimensions=[9]  SampleTime=1e-08
  globalSchedule : EnablePort  OutDataTypeStr=boolean
  PipelineRegister : Delay  DelayLength=double(8)  InitialCondition=0
  t : hdlsllib/HDL Operations/Multiply-Accumulate  opMode=Vector  initValueSetting=Dialog  initValue=0  initValueSetting2=Dialog  initValue2=0  initValueSetting3=Dialog  initValue3=0  num_samples=2  RndMeth2=Floor  RndMeth3=Floor  OutDataTypeStr=fixdt(1, 25, 12)  datatype2=Inherit: Inherit via back propagation  datatype3=Inherit: Inherit via back propagation  validOut=on  endInandOut=on  startOut=on  countOut=on  dim=-1  DoSatur=off  parallel=off
      settings: SourceProductBaseCode=SL
  out0 : Outport  OutDataTypeStr=fixdt(1, 25, 12)  SampleTime=1e-08  InitialOutput=0
  wires:
  t/1 -> PipelineRegister/1
  in1/1 -> t/2
  in0/1 -> t/1
  PipelineRegister/1 -> out0/1

== system gm_uz_pmsm_model_9ph_21b_all_double_vnl/uz_pmsm_model_9ph/Transformation1/Transformation1_MAC6 ==
  in0 : Inport  OutDataTypeStr=fixdt(1, 18, 16)  PortDimensions=[9 1]  SampleTime=1e-08
  in1 : Inport  Port=2  OutDataTypeStr=fixdt(1, 25, 12)  PortDimensions=[9]  SampleTime=1e-08
  globalSchedule : EnablePort  OutDataTypeStr=boolean
  PipelineRegister : Delay  DelayLength=double(8)  InitialCondition=0
  t : hdlsllib/HDL Operations/Multiply-Accumulate  opMode=Vector  initValueSetting=Dialog  initValue=0  initValueSetting2=Dialog  initValue2=0  initValueSetting3=Dialog  initValue3=0  num_samples=2  RndMeth2=Floor  RndMeth3=Floor  OutDataTypeStr=fixdt(1, 25, 12)  datatype2=Inherit: Inherit via back propagation  datatype3=Inherit: Inherit via back propagation  validOut=on  endInandOut=on  startOut=on  countOut=on  dim=-1  DoSatur=off  parallel=off
      settings: SourceProductBaseCode=SL
  out0 : Outport  OutDataTypeStr=fixdt(1, 25, 12)  SampleTime=1e-08  InitialOutput=0
  wires:
  t/1 -> PipelineRegister/1
  in1/1 -> t/2
  in0/1 -> t/1
  PipelineRegister/1 -> out0/1

== system gm_uz_pmsm_model_9ph_21b_all_double_vnl/uz_pmsm_model_9ph/Transformation1/Transformation1_MAC7 ==
  in0 : Inport  OutDataTypeStr=fixdt(1, 18, 16)  PortDimensions=[9 1]  SampleTime=1e-08
  in1 : Inport  Port=2  OutDataTypeStr=fixdt(1, 25, 12)  PortDimensions=[9]  SampleTime=1e-08
  globalSchedule : EnablePort  OutDataTypeStr=boolean
  PipelineRegister : Delay  DelayLength=double(8)  InitialCondition=0
  t : hdlsllib/HDL Operations/Multiply-Accumulate  opMode=Vector  initValueSetting=Dialog  initValue=0  initValueSetting2=Dialog  initValue2=0  initValueSetting3=Dialog  initValue3=0  num_samples=2  RndMeth2=Floor  RndMeth3=Floor  OutDataTypeStr=fixdt(1, 25, 12)  datatype2=Inherit: Inherit via back propagation  datatype3=Inherit: Inherit via back propagation  validOut=on  endInandOut=on  startOut=on  countOut=on  dim=-1  DoSatur=off  parallel=off
      settings: SourceProductBaseCode=SL
  out0 : Outport  OutDataTypeStr=fixdt(1, 25, 12)  SampleTime=1e-08  InitialOutput=0
  wires:
  t/1 -> PipelineRegister/1
  in1/1 -> t/2
  in0/1 -> t/1
  PipelineRegister/1 -> out0/1

== system gm_uz_pmsm_model_9ph_21b_all_double_vnl/uz_pmsm_model_9ph/Transformation1/Transformation1_MAC8 ==
  in0 : Inport  OutDataTypeStr=fixdt(1, 18, 16)  PortDimensions=[9 1]  SampleTime=1e-08
  in1 : Inport  Port=2  OutDataTypeStr=fixdt(1, 25, 12)  PortDimensions=[9]  SampleTime=1e-08
  globalSchedule : EnablePort  OutDataTypeStr=boolean
  PipelineRegister : Delay  DelayLength=double(8)  InitialCondition=0
  t : hdlsllib/HDL Operations/Multiply-Accumulate  opMode=Vector  initValueSetting=Dialog  initValue=0  initValueSetting2=Dialog  initValue2=0  initValueSetting3=Dialog  initValue3=0  num_samples=2  RndMeth2=Floor  RndMeth3=Floor  OutDataTypeStr=fixdt(1, 25, 12)  datatype2=Inherit: Inherit via back propagation  datatype3=Inherit: Inherit via back propagation  validOut=on  endInandOut=on  startOut=on  countOut=on  dim=-1  DoSatur=off  parallel=off
      settings: SourceProductBaseCode=SL
  out0 : Outport  OutDataTypeStr=fixdt(1, 25, 12)  SampleTime=1e-08  InitialOutput=0
  wires:
  t/1 -> PipelineRegister/1
  in1/1 -> t/2
  in0/1 -> t/1
  PipelineRegister/1 -> out0/1

== system gm_uz_pmsm_model_9ph_21b_all_double_vnl/uz_pmsm_model_9ph/Transformation1/t3 ==
  in0 : Inport
  ColVec1 : Selector  NumberOfDimensions=2  IndexOptions=Select all,Index vector (dialog)  Indices=1,1  OutputSizes=1,1
  ColVec2 : Selector  NumberOfDimensions=2  IndexOptions=Select all,Index vector (dialog)  Indices=1,2  OutputSizes=1,1
  ColVec3 : Selector  NumberOfDimensions=2  IndexOptions=Select all,Index vector (dialog)  Indices=1,3  OutputSizes=1,1
  ColVec4 : Selector  NumberOfDimensions=2  IndexOptions=Select all,Index vector (dialog)  Indices=1,4  OutputSizes=1,1
  ColVec5 : Selector  NumberOfDimensions=2  IndexOptions=Select all,Index vector (dialog)  Indices=1,5  OutputSizes=1,1
  ColVec6 : Selector  NumberOfDimensions=2  IndexOptions=Select all,Index vector (dialog)  Indices=1,6  OutputSizes=1,1
  ColVec7 : Selector  NumberOfDimensions=2  IndexOptions=Select all,Index vector (dialog)  Indices=1,7  OutputSizes=1,1
  ColVec8 : Selector  NumberOfDimensions=2  IndexOptions=Select all,Index vector (dialog)  Indices=1,8  OutputSizes=1,1
  ColVec9 : Selector  NumberOfDimensions=2  IndexOptions=Select all,Index vector (dialog)  Indices=1,9  OutputSizes=1,1
  out0 : Outport
  out1 : Outport  Port=2
  out2 : Outport  Port=3
  out3 : Outport  Port=4
  out4 : Outport  Port=5
  out5 : Outport  Port=6
  out6 : Outport  Port=7
  out7 : Outport  Port=8
  out8 : Outport  Port=9
  wires:
  ColVec9/1 -> out8/1
  ColVec8/1 -> out7/1
  ColVec7/1 -> out6/1
  ColVec6/1 -> out5/1
  ColVec5/1 -> out4/1
  ColVec4/1 -> out3/1
  ColVec3/1 -> out2/1
  ColVec2/1 -> out1/1
  ColVec1/1 -> out0/1
  in0/1 -> ColVec9/1, ColVec8/1, ColVec7/1, ColVec6/1, ColVec5/1, ColVec4/1, ColVec3/1, ColVec2/1, ColVec1/1

== system gm_uz_pmsm_model_9ph_21b_all_double_vnl/uz_pmsm_model_9ph/dq_model_9ph/Add ==
  In1 : Inport
  In2 : Inport  Port=2
  Add : Sum  Inputs=+-  OutDataTypeStr=double  SampleTime=1e-08
  Add_pd1 : Delay  DelayLength=6
  Out1 : Outport
  wires:
  Add_pd1/1 -> Out1/1
  Add/1 -> Add_pd1/1
  In2/1 -> Add/2
  In1/1 -> Add/1

== system gm_uz_pmsm_model_9ph_21b_all_double_vnl/uz_pmsm_model_9ph/dq_model_9ph/Add1 ==
  In1 : Inport
  In2 : Inport  Port=2
  Add1 : Sum  Inputs=+-  OutDataTypeStr=double  SampleTime=1e-08
  Add1_pd1 : Delay  DelayLength=6
  Out1 : Outport
  wires:
  Add1_pd1/1 -> Out1/1
  Add1/1 -> Add1_pd1/1
  In2/1 -> Add1/2
  In1/1 -> Add1/1

== system gm_uz_pmsm_model_9ph_21b_all_double_vnl/uz_pmsm_model_9ph/dq_model_9ph/Add2 ==
  In1 : Inport
  In2 : Inport  Port=2
  Add2 : Sum  Inputs=+-  OutDataTypeStr=double  SampleTime=1e-08
  Add2_pd1 : Delay  DelayLength=6
  Out1 : Outport
  wires:
  Add2_pd1/1 -> Out1/1
  Add2/1 -> Add2_pd1/1
  In2/1 -> Add2/2
  In1/1 -> Add2/1

== system gm_uz_pmsm_model_9ph_21b_all_double_vnl/uz_pmsm_model_9ph/dq_model_9ph/Add3 ==
  In1 : Inport
  In2 : Inport  Port=2
  Add3 : Sum  Inputs=+-  OutDataTypeStr=double  SampleTime=1e-08
  Add3_pd1 : Delay  DelayLength=6
  Out1 : Outport
  wires:
  Add3_pd1/1 -> Out1/1
  Add3/1 -> Add3_pd1/1
  In2/1 -> Add3/2
  In1/1 -> Add3/1

== system gm_uz_pmsm_model_9ph_21b_all_double_vnl/uz_pmsm_model_9ph/dq_model_9ph/Add4 ==
  In1 : Inport
  In2 : Inport  Port=2
  Add4 : Sum  Inputs=+-  OutDataTypeStr=double  SampleTime=1e-08
  Add4_pd1 : Delay  DelayLength=6
  Out1 : Outport
  wires:
  Add4_pd1/1 -> Out1/1
  Add4/1 -> Add4_pd1/1
  In2/1 -> Add4/2
  In1/1 -> Add4/1

== system gm_uz_pmsm_model_9ph_21b_all_double_vnl/uz_pmsm_model_9ph/dq_model_9ph/Add5 ==
  In1 : Inport
  In2 : Inport  Port=2
  Add5 : Sum  Inputs=+-  OutDataTypeStr=double  SampleTime=1e-08
  Add5_pd1 : Delay  DelayLength=6
  Out1 : Outport
  wires:
  Add5_pd1/1 -> Out1/1
  Add5/1 -> Add5_pd1/1
  In2/1 -> Add5/2
  In1/1 -> Add5/1

== system gm_uz_pmsm_model_9ph_21b_all_double_vnl/uz_pmsm_model_9ph/dq_model_9ph/Add6 ==
  In1 : Inport
  In2 : Inport  Port=2
  Add6 : Sum  Inputs=+-  OutDataTypeStr=double  SampleTime=1e-08
  Add6_pd1 : Delay  DelayLength=6
  Out1 : Outport
  wires:
  Add6_pd1/1 -> Out1/1
  Add6/1 -> Add6_pd1/1
  In2/1 -> Add6/2
  In1/1 -> Add6/1

== system gm_uz_pmsm_model_9ph_21b_all_double_vnl/uz_pmsm_model_9ph/dq_model_9ph/Compare To Constant1_relop ==
  In1 : Inport
  In2 : Inport  Port=2
  Compare To Constant1_relop : RelationalOperator  Operator=<  OutDataTypeStr=boolean  SampleTime=1e-08  RndMeth=Nearest  InputSameDT=on
  Compare To Constant1_relop_pd1 : Delay  DelayLength=1
  Out1 : Outport
  wires:
  Compare To Constant1_relop_pd1/1 -> Out1/1
  Compare To Constant1_relop/1 -> Compare To Constant1_relop_pd1/1
  In2/1 -> Compare To Constant1_relop/2
  In1/1 -> Compare To Constant1_relop/1

== system gm_uz_pmsm_model_9ph_21b_all_double_vnl/uz_pmsm_model_9ph/dq_model_9ph/Compare To Constant_relop ==
  In1 : Inport
  In2 : Inport  Port=2
  Compare To Constant_relop : RelationalOperator  OutDataTypeStr=boolean  SampleTime=1e-08  RndMeth=Nearest  InputSameDT=on
  Compare To Constant_relop_pd1 : Delay  DelayLength=1
  Out1 : Outport
  wires:
  Compare To Constant_relop_pd1/1 -> Out1/1
  Compare To Constant_relop/1 -> Compare To Constant_relop_pd1/1
  In2/1 -> Compare To Constant_relop/2
  In1/1 -> Compare To Constant_relop/1

== system gm_uz_pmsm_model_9ph_21b_all_double_vnl/uz_pmsm_model_9ph/dq_model_9ph/Data Type Conversion ==
  In1 : Inport
  Data Type Conversion : DataTypeConversion  OutDataTypeStr=double  RndMeth=Nearest  SampleTime=1e-08
  Data Type Conversion_pd1 : Delay  DelayLength=3
  Out1 : Outport
  wires:
  Data Type Conversion_pd1/1 -> Out1/1
  Data Type Conversion/1 -> Data Type Conversion_pd1/1
  In1/1 -> Data Type Conversion/1

== system gm_uz_pmsm_model_9ph_21b_all_double_vnl/uz_pmsm_model_9ph/dq_model_9ph/Data Type Conversion1 ==
  In1 : Inport
  Data Type Conversion1 : DataTypeConversion  OutDataTypeStr=double  RndMeth=Nearest  SampleTime=1e-08
  Data Type Conversion1_pd1 : Delay  DelayLength=3
  Out1 : Outport
  wires:
  Data Type Conversion1_pd1/1 -> Out1/1
  Data Type Conversion1/1 -> Data Type Conversion1_pd1/1
  In1/1 -> Data Type Conversion1/1

== system gm_uz_pmsm_model_9ph_21b_all_double_vnl/uz_pmsm_model_9ph/dq_model_9ph/Data Type Conversion10 ==
  In1 : Inport
  Data Type Conversion10 : DataTypeConversion  OutDataTypeStr=double  RndMeth=Nearest  SampleTime=1e-08
  Data Type Conversion10_pd1 : Delay  DelayLength=3
  Out1 : Outport
  wires:
  Data Type Conversion10_pd1/1 -> Out1/1
  Data Type Conversion10/1 -> Data Type Conversion10_pd1/1
  In1/1 -> Data Type Conversion10/1

== system gm_uz_pmsm_model_9ph_21b_all_double_vnl/uz_pmsm_model_9ph/dq_model_9ph/Data Type Conversion11 ==
  In1 : Inport
  Data Type Conversion11 : DataTypeConversion  OutDataTypeStr=double  RndMeth=Nearest  SampleTime=1e-08
  Data Type Conversion11_pd1 : Delay  DelayLength=3
  Out1 : Outport
  wires:
  Data Type Conversion11_pd1/1 -> Out1/1
  Data Type Conversion11/1 -> Data Type Conversion11_pd1/1
  In1/1 -> Data Type Conversion11/1

== system gm_uz_pmsm_model_9ph_21b_all_double_vnl/uz_pmsm_model_9ph/dq_model_9ph/Data Type Conversion12 ==
  In1 : Inport
  Data Type Conversion12 : DataTypeConversion  OutDataTypeStr=double  RndMeth=Nearest  SampleTime=1e-08
  Data Type Conversion12_pd1 : Delay  DelayLength=3
  Out1 : Outport
  wires:
  Data Type Conversion12_pd1/1 -> Out1/1
  Data Type Conversion12/1 -> Data Type Conversion12_pd1/1
  In1/1 -> Data Type Conversion12/1

== system gm_uz_pmsm_model_9ph_21b_all_double_vnl/uz_pmsm_model_9ph/dq_model_9ph/Data Type Conversion13 ==
  In1 : Inport
  Data Type Conversion13 : DataTypeConversion  OutDataTypeStr=double  RndMeth=Nearest  SampleTime=1e-08
  Data Type Conversion13_pd1 : Delay  DelayLength=3
  Out1 : Outport
  wires:
  Data Type Conversion13_pd1/1 -> Out1/1
  Data Type Conversion13/1 -> Data Type Conversion13_pd1/1
  In1/1 -> Data Type Conversion13/1

== system gm_uz_pmsm_model_9ph_21b_all_double_vnl/uz_pmsm_model_9ph/dq_model_9ph/Data Type Conversion2 ==
  In1 : Inport
  Data Type Conversion2 : DataTypeConversion  OutDataTypeStr=double  RndMeth=Nearest  SampleTime=1e-08
  Data Type Conversion2_pd1 : Delay  DelayLength=3
  Out1 : Outport
  wires:
  Data Type Conversion2_pd1/1 -> Out1/1
  Data Type Conversion2/1 -> Data Type Conversion2_pd1/1
  In1/1 -> Data Type Conversion2/1

== system gm_uz_pmsm_model_9ph_21b_all_double_vnl/uz_pmsm_model_9ph/dq_model_9ph/Data Type Conversion21 ==
  In1 : Inport
  Data Type Conversion21 : DataTypeConversion  OutDataTypeStr=double  RndMeth=Nearest  SampleTime=1e-08
  Data Type Conversion21_pd1 : Delay  DelayLength=3
  Out1 : Outport
  wires:
  Data Type Conversion21_pd1/1 -> Out1/1
  Data Type Conversion21/1 -> Data Type Conversion21_pd1/1
  In1/1 -> Data Type Conversion21/1

== system gm_uz_pmsm_model_9ph_21b_all_double_vnl/uz_pmsm_model_9ph/dq_model_9ph/Data Type Conversion3 ==
  In1 : Inport
  Data Type Conversion3 : DataTypeConversion  OutDataTypeStr=single  RndMeth=Nearest  SampleTime=1e-08
  Data Type Conversion3_pd1 : Delay  DelayLength=3
  Out1 : Outport
  wires:
  Data Type Conversion3_pd1/1 -> Out1/1
  Data Type Conversion3/1 -> Data Type Conversion3_pd1/1
  In1/1 -> Data Type Conversion3/1

== system gm_uz_pmsm_model_9ph_21b_all_double_vnl/uz_pmsm_model_9ph/dq_model_9ph/Data Type Conversion31 ==
  In1 : Inport
  Data Type Conversion31 : DataTypeConversion  OutDataTypeStr=double  RndMeth=Nearest  SampleTime=1e-08
  Data Type Conversion31_pd1 : Delay  DelayLength=3
  Out1 : Outport
  wires:
  Data Type Conversion31_pd1/1 -> Out1/1
  Data Type Conversion31/1 -> Data Type Conversion31_pd1/1
  In1/1 -> Data Type Conversion31/1

== system gm_uz_pmsm_model_9ph_21b_all_double_vnl/uz_pmsm_model_9ph/dq_model_9ph/Data Type Conversion4 ==
  In1 : Inport
  Data Type Conversion4 : DataTypeConversion  OutDataTypeStr=single  RndMeth=Nearest  SampleTime=1e-08
  Data Type Conversion4_pd1 : Delay  DelayLength=3
  Out1 : Outport
  wires:
  Data Type Conversion4_pd1/1 -> Out1/1
  Data Type Conversion4/1 -> Data Type Conversion4_pd1/1
  In1/1 -> Data Type Conversion4/1

== system gm_uz_pmsm_model_9ph_21b_all_double_vnl/uz_pmsm_model_9ph/dq_model_9ph/Data Type Conversion41 ==
  In1 : Inport
  Data Type Conversion41 : DataTypeConversion  OutDataTypeStr=double  RndMeth=Nearest  SampleTime=1e-08
  Data Type Conversion41_pd1 : Delay  DelayLength=3
  Out1 : Outport
  wires:
  Data Type Conversion41_pd1/1 -> Out1/1
  Data Type Conversion41/1 -> Data Type Conversion41_pd1/1
  In1/1 -> Data Type Conversion41/1

== system gm_uz_pmsm_model_9ph_21b_all_double_vnl/uz_pmsm_model_9ph/dq_model_9ph/Data Type Conversion5 ==
  In1 : Inport
  Data Type Conversion5 : DataTypeConversion  OutDataTypeStr=single  RndMeth=Nearest  SampleTime=1e-08
  Data Type Conversion5_pd1 : Delay  DelayLength=3
  Out1 : Outport
  wires:
  Data Type Conversion5_pd1/1 -> Out1/1
  Data Type Conversion5/1 -> Data Type Conversion5_pd1/1
  In1/1 -> Data Type Conversion5/1

== system gm_uz_pmsm_model_9ph_21b_all_double_vnl/uz_pmsm_model_9ph/dq_model_9ph/Data Type Conversion51 ==
  In1 : Inport
  Data Type Conversion51 : DataTypeConversion  OutDataTypeStr=double  RndMeth=Nearest  SampleTime=1e-08
  Data Type Conversion51_pd1 : Delay  DelayLength=3
  Out1 : Outport
  wires:
  Data Type Conversion51_pd1/1 -> Out1/1
  Data Type Conversion51/1 -> Data Type Conversion51_pd1/1
  In1/1 -> Data Type Conversion51/1

== system gm_uz_pmsm_model_9ph_21b_all_double_vnl/uz_pmsm_model_9ph/dq_model_9ph/Data Type Conversion6 ==
  In1 : Inport
  Data Type Conversion6 : DataTypeConversion  OutDataTypeStr=single  RndMeth=Nearest  SampleTime=1e-08
  Data Type Conversion6_pd1 : Delay  DelayLength=3
  Out1 : Outport
  wires:
  Data Type Conversion6_pd1/1 -> Out1/1
  Data Type Conversion6/1 -> Data Type Conversion6_pd1/1
  In1/1 -> Data Type Conversion6/1

== system gm_uz_pmsm_model_9ph_21b_all_double_vnl/uz_pmsm_model_9ph/dq_model_9ph/Data Type Conversion61 ==
  In1 : Inport
  Data Type Conversion61 : DataTypeConversion  OutDataTypeStr=double  RndMeth=Nearest  SampleTime=1e-08
  Data Type Conversion61_pd1 : Delay  DelayLength=3
  Out1 : Outport
  wires:
  Data Type Conversion61_pd1/1 -> Out1/1
  Data Type Conversion61/1 -> Data Type Conversion61_pd1/1
  In1/1 -> Data Type Conversion61/1
